simulink model "Example_R2025b"  (R2025b)
settings: Solver=VariableStepAuto  StartTime=0.0  StopTime=100  RelTol=1e-3
libraries: ForceSeatDI_Simulink_R2025b x3
settings Model: Creator=usr  LastModifiedBy=WDAGUtilityAccount
settings SolverCC: AlgebraicLoopSolver=TrustRegion
settings DebuggingCC: UnconnectedInputMsg=warning  UnconnectedOutputMsg=warning  UnconnectedLineMsg=warning
settings ModelReferenceCC: EnableRefExpFcnMdlSchedulingChecks=on
settings RTWCC: GPUComputeCapability=3.5

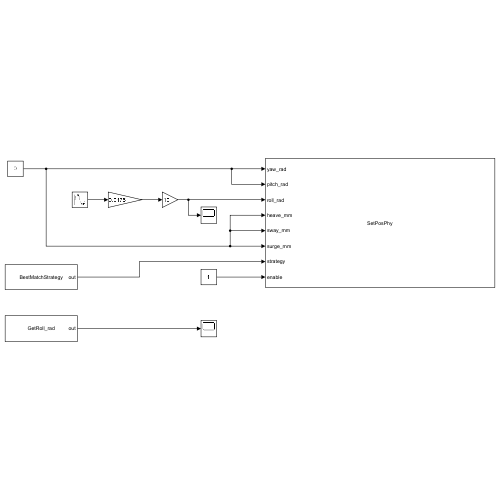
[thumbnail: Simulink's stored preview of the top-level diagram]
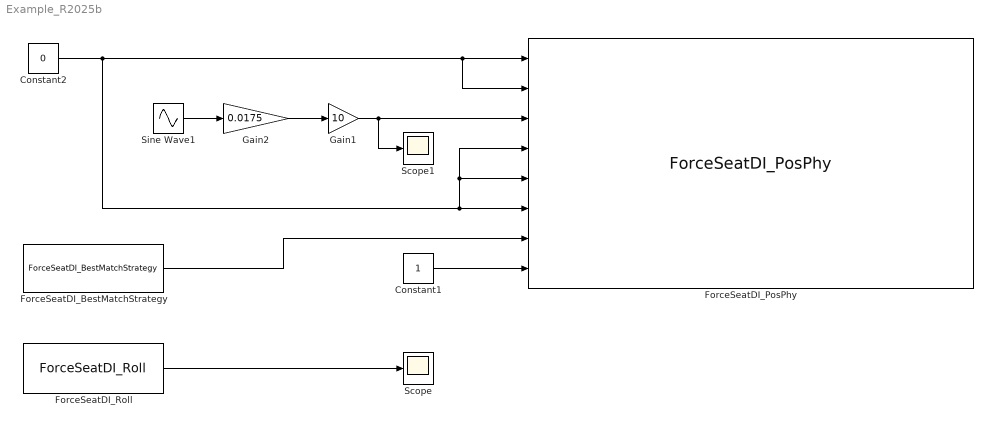
== system Example_R2025b ==
  Constant1 : Constant  OutDataTypeStr=int32
  Constant2 : Constant  Value=0
  ForceSeatDI_BestMatchStrategy : ForceSeatDI_Simulink_R2025b/ForceSeatDI_BestMatchStrategy  SampleTime=-1
  ForceSeatDI_PosPhy : ForceSeatDI_Simulink_R2025b/ForceSeatDI_PosPhy  SampleTime=-1
      settings: SourceProductName=MotionSystems ForceSeatDI R2025b
  ForceSeatDI_Roll : ForceSeatDI_Simulink_R2025b/ForceSeatDI_Roll  SampleTime=-1
      settings: SourceProductName=MotionSystems ForceSeatDI R2025b
  Gain1 : Gain  Gain=10
  Gain2 : Gain  Gain=0.0175
  Scope : Scope
  Scope1 : Scope
      settings: ActiveDisplayYMinimum=-0.21875  ActiveDisplayYMaximum=0.21875
  Sine Wave1 : Sin  SampleTime=0.01
  wires:
  Constant1/1 -> ForceSeatDI_PosPhy/8
  Constant2/1 -> ForceSeatDI_PosPhy/2, ForceSeatDI_PosPhy/1, ForceSeatDI_PosPhy/6, ForceSeatDI_PosPhy/4, ForceSeatDI_PosPhy/5
  Sine Wave1/1 -> Gain2/1
  Gain2/1 -> Gain1/1
  Gain1/1 -> ForceSeatDI_PosPhy/3, Scope1/1
  ForceSeatDI_Roll/1 -> Scope/1
  ForceSeatDI_BestMatchStrategy/1 -> ForceSeatDI_PosPhy/7
